simulink model "ApplBTA_LDM"  (R2018b)
settings: Solver=FixedStepAuto  StartTime=0.0  StopTime=10.0  FixedStep=0.002  RelTol=1e-3
libraries: LDM_Controller x1
settings Model: DataDictionary=totalDataDict.sldd  Creator=wxmjy  LastModifiedBy=wxmjy
settings OptimizationCC: DefaultParameterBehavior=Inlined  EnhancedBackFolding=on  PassReuseOutputArgsAs=Individual arguments  OptimizeBlockOrder=speed  DifferentSizesBufferReuse=on  OptimizationCustomize=off
settings DebuggingCC: ParameterTunabilityLossMsg=error
settings SFSimCC: MATLABDynamicMemAlloc=off
settings RTWCC: SystemTargetFile=ert.tlc  GenCodeOnly=on  TemplateMakefile=ert_default_tmf  GenerateReport=on  IncludeHyperlinkInReport=on  LaunchReport=on  GenerateTraceInfo=on  GenerateTraceReport=on  GenerateTraceReportSl=on  GenerateTraceReportSf=on  GenerateTraceReportEml=on
settings CodeAppCC: ForceParamTrailComments=on  IgnoreCustomStorageClasses=off  OperatorAnnotations=on  SimulinkDataObjDesc=on  SFDataObjDesc=on  InsertBlockDesc=on
settings ERTTargetCC: TargetLangStandard=C99 (ISO)  GenerateSampleERTMain=on  SupportComplex=off  GenerateASAP2=on  InlinedParameterPlacement=NonHierarchical  ERTCustomFileTemplate=example_file_process.tlc  EnableUserReplacementTypes=on

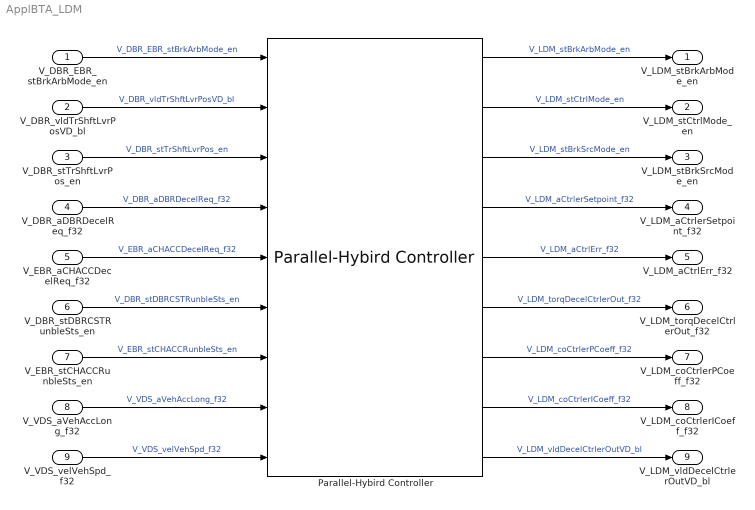
== system ApplBTA_LDM ==
  V_DBR_EBR_stBrkArbMode_en : Inport
  V_DBR_vldTrShftLvrPosVD_bl : Inport  Port=2
  V_DBR_stTrShftLvrPos_en : Inport  Port=3
  V_DBR_aDBRDecelReq_f32 : Inport  Port=4
  V_EBR_aCHACCDecelReq_f32 : Inport  Port=5
  V_DBR_stDBRCSTRunbleSts_en : Inport  Port=6
  V_EBR_stCHACCRunbleSts_en : Inport  Port=7
  V_VDS_aVehAccLong_f32 : Inport  Port=8
  V_VDS_velVehSpd_f32 : Inport  Port=9
  Parallel-Hybird Controller : LDM_Controller/Parallel-Hybird Controller  SystemSampleTime=-1
  V_LDM_stBrkArbMode_en : Outport
  V_LDM_stCtrlMode_en : Outport  Port=2
  V_LDM_stBrkSrcMode_en : Outport  Port=3
  V_LDM_aCtrlerSetpoint_f32 : Outport  Port=4
  V_LDM_aCtrlErr_f32 : Outport  Port=5
  V_LDM_torqDecelCtrlerOut_f32 : Outport  Port=6
  V_LDM_coCtrlerPCoeff_f32 : Outport  Port=7
  V_LDM_coCtrlerICoeff_f32 : Outport  Port=8
  V_LDM_vldDecelCtrlerOutVD_bl : Outport  Port=9
  wires:
  V_DBR_EBR_stBrkArbMode_en/1 -> Parallel-Hybird Controller/1  "V_DBR_EBR_stBrkArbMode_en"
  V_DBR_vldTrShftLvrPosVD_bl/1 -> Parallel-Hybird Controller/2  "V_DBR_vldTrShftLvrPosVD_bl"
  V_DBR_stTrShftLvrPos_en/1 -> Parallel-Hybird Controller/3  "V_DBR_stTrShftLvrPos_en"
  V_DBR_aDBRDecelReq_f32/1 -> Parallel-Hybird Controller/4  "V_DBR_aDBRDecelReq_f32"
  V_EBR_aCHACCDecelReq_f32/1 -> Parallel-Hybird Controller/5  "V_EBR_aCHACCDecelReq_f32"
  V_DBR_stDBRCSTRunbleSts_en/1 -> Parallel-Hybird Controller/6  "V_DBR_stDBRCSTRunbleSts_en"
  V_EBR_stCHACCRunbleSts_en/1 -> Parallel-Hybird Controller/7  "V_EBR_stCHACCRunbleSts_en"
  V_VDS_aVehAccLong_f32/1 -> Parallel-Hybird Controller/8  "V_VDS_aVehAccLong_f32"
  V_VDS_velVehSpd_f32/1 -> Parallel-Hybird Controller/9  "V_VDS_velVehSpd_f32"
  Parallel-Hybird Controller/1 -> V_LDM_stBrkArbMode_en/1  "V_LDM_stBrkArbMode_en"
  Parallel-Hybird Controller/2 -> V_LDM_stCtrlMode_en/1  "V_LDM_stCtrlMode_en"
  Parallel-Hybird Controller/3 -> V_LDM_stBrkSrcMode_en/1  "V_LDM_stBrkSrcMode_en"
  Parallel-Hybird Controller/4 -> V_LDM_aCtrlerSetpoint_f32/1  "V_LDM_aCtrlerSetpoint_f32"
  Parallel-Hybird Controller/5 -> V_LDM_aCtrlErr_f32/1  "V_LDM_aCtrlErr_f32"
  Parallel-Hybird Controller/6 -> V_LDM_torqDecelCtrlerOut_f32/1  "V_LDM_torqDecelCtrlerOut_f32"
  Parallel-Hybird Controller/7 -> V_LDM_coCtrlerPCoeff_f32/1  "V_LDM_coCtrlerPCoeff_f32"
  Parallel-Hybird Controller/8 -> V_LDM_coCtrlerICoeff_f32/1  "V_LDM_coCtrlerICoeff_f32"
  Parallel-Hybird Controller/9 -> V_LDM_vldDecelCtrlerOutVD_bl/1  "V_LDM_vldDecelCtrlerOutVD_bl"
